simulink model "GTA_PCMFirmware"  (Simulink 7.8)
settings: Solver=FixedStepDiscrete  StartTime=0.0  StopTime=10.0  RelTol=1e-3
PreLoadFcn:
  | try, eval([bdroot '_setup']); catch, eval('model_setup', ''); end
InitFcn:
  | try, eval([bdroot '_setup']); catch, eval('model_setup', ''); end
undefined symbols (not defined in the file): fndFwd, fndNeut, fndRev, FWDlockout, GCM, keySwIgn2, motohawk_build_version, motohawk_trunc_name, motohawk_vardec_path, REVlockout
libraries: MotoHawk_lib x313, simulink x47, GTA_Library x13
(part 7 of 7)

== stateflow chart Function/2 Control Loop/Mode Control & Ready/Mode Control/Mode Control ==
  state ModeControl [parallel]
    settings: executionOrder=1
    state RUN
      state Drive
        en:
        ModeState = 5;
        HVmode = 3;
      state Startup
        en:
        ModeState = 0;
        HVmode = 0;
        ChargeEnable = 0;
      state Charge
        en:
        ModeState = 1;
        HVmode = 2;
        ChargeEnable = 1;
      state ChargeAndACC
        en:
        ModeState = 2;
        HVmode = 2;
        ChargeEnable = 1;
      state ACC1
        en:
        ModeState = 3;
        HVmode = 0;
        ChargeEnable = 0;
      state ACC2
        en:
        ModeState = 4;
        HVmode = 1;
      Startup -> Charge [order 1] : [acPresent == 1]
      (default) -> Startup
      Charge -> ChargeAndACC [order 1] : [keySw > 0]
      ChargeAndACC -> Charge [order 1] : [keySw == 0]
      Startup -> ACC1 [order 2] : [keySw > 0]
      ACC1 -> Startup [order 1] : [keySw == 0]
      ChargeAndACC -> ACC1 [order 2] : [acPresent == 0]
      ACC1 -> ChargeAndACC [order 2] : [acPresent == 1]
      ACC1 -> ACC2 [order 3] : [keySw > 1]
      ACC2 -> ACC1 [order 1] : [keySw < 2]
      ACC2 -> Drive [order 2] : [Ready == 1 && keySw == 6]
      Drive -> ACC1 [order 1] : [keySw < 2]
      ACC2 -> ChargeAndACC [order 3] : [acPresent == 1]
      Drive -> ChargeAndACC [order 2] : [acPresent == 1]
      Charge -> Startup [order 2] : [acPresent == 0]
    state Inhibit
      en:
      ModeState = 7;
      ChargeEnable = 0;
      HVmode = 0;
    RUN -> Inhibit : SysFault
    (default) -> RUN
  state HVControl [parallel]
    settings: executionOrder=2
    state Mode0
      en:
      HVstate = 0;
      SSCont = 0;
      MainCont = 0;
      HVaccRly = 0;
      DriveOn = 0;
    state DriveOn
      en:
      HVstate = 1;
      SSCont = 1;
      MainCont = 0;
      HVaccRly = 0;
      DriveOn = 0;
    state Limbo
    state PreCharge
      en:
      HVstate = 2;
      SSCont = 1;
      MainCont = 0;
      HVaccRly = 0;
      DriveOn = 1;
    state PreCharge2
      en:
      HVstate = 3;
      SSCont = 1;
      MainCont = 1;
      HVaccRly = 0;
      DriveOn = 1;
    state Mode1
      en:
      HVstate = 4;
      SSCont = 1;
      MainCont = 1;
      HVaccRly = 0;
      DriveOn = 0;
    state Mode3
      en:
      HVstate = 8;
      SSCont = 1;
      MainCont = 1;
      HVaccRly = 1;
      DriveOn = 1;
    state Mode2
      en:
      HVstate = 5;
      SSCont = 0;
      MainCont = 1;
      HVaccRly = 1;
      DriveOn = 0;
    state DriveDisable
      en:
      HVstate = 7;
      SSCont = 0;
      MainCont = 1;
      HVaccRly = 0;
      DriveOn = 0;
    state Startup_PauseHV
      en:
      HVstate = 0;
      SSCont = 0;
      MainCont = 0;
      HVaccRly = 0;
      DriveOn = 0
    Mode0 -> HVControl.DriveOn : [HVmode > 0]
    HVControl.DriveOn -> Mode0 [order 1] : [HVmode == 0]
    HVControl.DriveOn -> Limbo [order 2] : [VoltDiffPercent < 25]
    Limbo -> (junction 36) [order 1] : after(1000, tick) /send (ContFault);
    HVControl.DriveOn -> PreCharge [order 3] : after(100, tick)
    Limbo -> PreCharge [order 2] : [VoltDiffPercent > 25]
    (junction 37) -> (junction 36)
    PreCharge -> (junction 37) [order 1] : after(1000, tick) /send (PreChargeFault);
    PreCharge -> PreCharge2 [order 2] : [VoltDiffPercent < 25]
    PreCharge2 -> (junction 37) [order 1] : [HVmode == 0]
    (junction 36) -> Mode0
    PreCharge2 -> Mode1 [order 2] : [HVmode == 1]
    PreCharge2 -> Mode1 [order 3] : [HVmode == 2]
    PreCharge2 -> Mode3 [order 4] : [HVmode == 3]
    Mode1 -> Mode3 [order 1] : [HVmode == 3]
    Mode1 -> Mode2 [order 2] : [HVmode == 2]
    Mode2 -> Mode1 [order 1] : [HVmode == 1]
    Mode2 -> Mode3 [order 2] : [HVmode == 3]
    Mode3 -> Mode2 [order 2] : [HVmode < 3]
    Mode1 -> (junction 38) [order 3] : [HVmode == 0]
    Mode2 -> (junction 38) [order 3] : [HVmode == 0]
    (junction 38) -> DriveDisable
    DriveDisable -> (junction 39) : after(20,tick)
    PreCharge -> (junction 39) [order 3] : [HVmode == 0]
    (junction 39) -> Mode0
    Mode3 -> Mode1 [order 1] : [HVmode == 1]
    (default) -> Startup_PauseHV
    Startup_PauseHV -> Mode0 : after(100, tick)
  state FaultControl [parallel]
    settings: executionOrder=4
    state eStop_Fault
      en:
      Fault_ID = 1;
    state Battery_Fault
      en:
      Fault_ID = 2;
    state Contactor_Fault
      en:
      Fault_ID = 4;
    state Startup_Pause
      en:
      Fault_ID = 0;
    state PreCharge_Fault
      en:
      Fault_ID = 5;
    state HVOff
      en:
      Fault_ID = 0;
    state Fault_Send
    state Fault_Sent
    HVOff -> eStop_Fault [order 1] : after(600, tick) [eStop == 1]
    HVOff -> Battery_Fault [order 2] : [BatteryFault > 0 && ChargeEnable == 0]
    Contactor_Fault -> Fault_Send
    HVOff -> Contactor_Fault [order 4] : ContFault
    HVOff -> PreCharge_Fault [order 3] : PreChargeFault
    eStop_Fault -> Fault_Send
    Battery_Fault -> Fault_Send
    (default) -> Startup_Pause
    Startup_Pause -> HVOff : after(200,tick)
    PreCharge_Fault -> Fault_Send
    Fault_Send -> Fault_Sent : /send (SysFault);
  state DriveControl [parallel]
    settings: executionOrder=3
    state HVoff
      en:
      DriveState = 0;
      DriveEnable = 0;
      MotorEnable = 0;
    state DriveOn
      en:
      DriveState = 1;
      DriveEnable = 1;
      MotorEnable = 0;
    state RuneMode
      en:
      DriveState = 2;
      DriveEnable = 1;
      MotorEnable = 1;
    (default) -> HVoff
    HVoff -> DriveControl.DriveOn : [DriveOn ==1]
    DriveControl.DriveOn -> HVoff [order 1] : [DriveOn == 0]
    DriveControl.DriveOn -> RuneMode [order 2] : [ModeState == 5 && HVstate == 8]
    RuneMode -> DriveControl.DriveOn : [ModeState ~= 5 || HVstate < 8]
  data: SSCont output boolean; MainCont output boolean; DriveEnable output boolean; HVaccRly output boolean; ModeState output uint8; ChargeEnable output boolean; HVstate output uint8; Fault_ID output uint8; DriveState output uint8; MotorEnable output boolean; HVmode local uint8; DriveOn local boolean; Ready input boolean; VoltageFault input boolean; BatteryFault input boolean; keySw input uint8; eStop input boolean; acPresent input boolean; VoltDiffPercent input single
  events: PreChargeFault local EITHER_EDGE_EVENT; ContFault local EITHER_EDGE_EVENT; SysFault local EITHER_EDGE_EVENT

== stateflow chart Function/2 Control Loop/Component Controls/Body Control/Defroster/Chart ==
  state Defroster_Off
    en:
    Defrost=0;
  state Switch_Release
  state Wait
    Defrost=0;
  state Defroster_On
    en:
    Defrost=1;
  (default) -> Defroster_Off
  Defroster_Off -> Switch_Release : [Defrost_sw==1]
  Defroster_On -> Wait [order 2] : after(60000,tick)
  Defroster_On -> Switch_Release [order 1] : after(200,tick) [Defrost_sw==1]
  Wait -> Defroster_Off : [Defrost_sw==0]
  Switch_Release -> Defroster_On : after(10,tick) [Defrost_sw==0]
  data: Defrost output boolean size=1; Defrost_sw input boolean size=1

== stateflow chart Function/2 Control Loop/Component Controls/Body Control/Inter Wiper/Chart ==
  state Calc
    en:
    Wiper_out=0;
  state Output_On
    en:
    Wiper_out=1;
  state State
    en:
    Time=200+(50*Pot_position);
    PotHi=Pot_position + 5;
    PotLo=Pot_position - 5;
  state Wiper_reset
  state Output_Off
    en:
    Wiper_out=0;
  Calc -> Output_On : [Wiper_Enable==1]
  Output_On -> Output_Off : after(200,tick)
  (default) -> Calc
  State -> Calc [order 1] : after(Time,tick)
  State -> Calc [order 2] : [Wiper_Enable==0]
  State -> Wiper_reset [order 3] : after(100,tick)[(Pot_position < PotLo) | (Pot_position > PotHi)]
  Wiper_reset -> Output_On
  Output_Off -> State : after(100,tick)
  data: Wiper_out output boolean size=1; Pot_position input single size=1; Time local uint32 size=1; Wiper_Enable input boolean size=1; PotLo local uint32 size=1; PotHi local uint32 size=1

== stateflow chart Function/2 Control Loop/Component Controls/Display Control/Fault Lamps/Red ErrorCodes ==
  state Error_Start
    en:
    Count = 0;
    State = 0;
    Error_out = 0;
  state Error3_Check
    state Error_Off
      en:
      Error_out=0;
    state Error_on
      en:
      Error_out = 1;
      Count = Count +1;
    state Error_en
      en:
      Count = 0;
    state Done
      en:
      State=3;
    Error3_Check.Error_Off -> Error3_Check.Done [order 2] : [Count >= Error3_blinks]
    Error3_Check.Error_on -> Error3_Check.Error_Off : after(150, tick)
    Error3_Check.Error_Off -> Error3_Check.Error_on [order 1] : after(150,tick)
    Error3_Check.Error_en -> Error3_Check.Error_on [order 2] : [Error3 ==1]
    (default) -> Error3_Check.Error_en
    Error3_Check.Error_en -> Error3_Check.Done [order 1] : [Error3 == 0]
  state Error2_Check
    state Error_Off
      en:
      Error_out=0;
    state Done
      en:
      State=2;
    state Error_on
      en:
      Error_out = 1;
      Count = Count +1;
    state Error_en
      en:
      Count = 0;
    Error2_Check.Error_Off -> Error2_Check.Error_on [order 1] : after(150,tick)
    Error2_Check.Error_Off -> Error2_Check.Done [order 2] : [Count >= Error2_blinks]
    Error2_Check.Error_on -> Error2_Check.Error_Off : after(150, tick)
    Error2_Check.Error_en -> Error2_Check.Done [order 1] : [Error2 == 0]
    Error2_Check.Error_en -> Error2_Check.Error_on [order 2] : [Error2 ==1]
    (default) -> Error2_Check.Error_en
  state Error1_Check
    state Error_en
      en:
      Count = 0;
    state Done
      en:
      State=1;
    state Error_on
      en:
      Error_out = 1;
      Count = Count +1;
    state Error_Off
      en:
      Error_out=0;
    (default) -> Error1_Check.Error_en
    Error1_Check.Error_en -> Error1_Check.Done [order 1] : [Error1 == 0]
    Error1_Check.Error_en -> Error1_Check.Error_on [order 2] : [Error1 ==1]
    Error1_Check.Error_Off -> Error1_Check.Done [order 2] : [Count >= Error1_blinks]
    Error1_Check.Error_Off -> Error1_Check.Error_on [order 1] : after(150,tick)
    Error1_Check.Error_on -> Error1_Check.Error_Off : after(150, tick)
  state Wait
  state Wait1
  state Wait2
  (default) -> Error_Start
  Error_Start -> Error1_Check
  Error1_Check -> Wait : [State==1]
  Error3_Check -> Wait2 : [State==3]
  Error2_Check -> Wait1 : [State==2]
  Wait -> Error2_Check : after(500,tick)
  Wait1 -> Error3_Check : after(500,tick)
  Wait2 -> Error_Start : after(500,tick)
  data: Error1 input double; Error1_blinks input double; Error2 input double; Error2_blinks input double; Error3 input double; Error3_blinks input double; Count output double; State output double; Error_out output boolean

== stateflow chart Function/2 Control Loop/Component Controls/Display Control/Fault Lamps/Yellow ErrorCodes ==
  state Error_Start
    en:
    Count = 0;
    State = 0;
    Error_out = 0;
  state Error3_Check
    state Error_Off
      en:
      Error_out=0;
    state Error_on
      en:
      Error_out = 1;
      Count = Count +1;
    state Error_en
      en:
      Count = 0;
    state Done
      en:
      State=3;
    Error3_Check.Error_Off -> Error3_Check.Done [order 2] : [Count >= Error3_blinks]
    Error3_Check.Error_on -> Error3_Check.Error_Off : after(150, tick)
    Error3_Check.Error_Off -> Error3_Check.Error_on [order 1] : after(150,tick)
    Error3_Check.Error_en -> Error3_Check.Error_on [order 2] : [Error3 ==1]
    (default) -> Error3_Check.Error_en
    Error3_Check.Error_en -> Error3_Check.Done [order 1] : [Error3 == 0]
  state Error2_Check
    state Error_Off
      en:
      Error_out=0;
    state Done
      en:
      State=2;
    state Error_on
      en:
      Error_out = 1;
      Count = Count +1;
    state Error_en
      en:
      Count = 0;
    Error2_Check.Error_Off -> Error2_Check.Error_on [order 1] : after(150,tick)
    Error2_Check.Error_Off -> Error2_Check.Done [order 2] : [Count >= Error2_blinks]
    Error2_Check.Error_on -> Error2_Check.Error_Off : after(150, tick)
    Error2_Check.Error_en -> Error2_Check.Done [order 1] : [Error2 == 0]
    Error2_Check.Error_en -> Error2_Check.Error_on [order 2] : [Error2 ==1]
    (default) -> Error2_Check.Error_en
  state Error1_Check
    state Error_en
      en:
      Count = 0;
    state Done
      en:
      State=1;
    state Error_on
      en:
      Error_out = 1;
      Count = Count +1;
    state Error_Off
      en:
      Error_out=0;
    (default) -> Error1_Check.Error_en
    Error1_Check.Error_en -> Error1_Check.Done [order 1] : [Error1 == 0]
    Error1_Check.Error_en -> Error1_Check.Error_on [order 2] : [Error1 ==1]
    Error1_Check.Error_Off -> Error1_Check.Done [order 2] : [Count >= Error1_blinks]
    Error1_Check.Error_Off -> Error1_Check.Error_on [order 1] : after(150,tick)
    Error1_Check.Error_on -> Error1_Check.Error_Off : after(150, tick)
  state Wait
  state Wait1
  state Wait2
  (default) -> Error_Start
  Error_Start -> Error1_Check
  Error1_Check -> Wait : [State==1]
  Error3_Check -> Wait2 : [State==3]
  Error2_Check -> Wait1 : [State==2]
  Wait -> Error2_Check : after(500,tick)
  Wait1 -> Error3_Check : after(500,tick)
  Wait2 -> Error_Start : after(500,tick)
  data: Error1 input double; Error1_blinks input double; Error2 input double; Error2_blinks input double; Error3 input double; Error3_blinks input double; Count output double; State output double; Error_out output boolean

== stateflow chart Function/2 Control Loop/Component Controls/Motor Control/Direction Selector & Control Loop/Rate Limiter Control Loop ==
  state Start
    Current_Out=0;
    ErrorAccum=0;
  state Error_calc
    error=Current_In - Current_Feedback;
  state Rising
    Current_Out = Current_Feedback + Rise;
  state Falling
    Current_Out = Current_Feedback + Fall;
  state Target
    Current_Out = Current_In;
  (default) -> Start
  Start -> Error_calc [order 2]
  Error_calc -> Rising [order 2] : [error > Rise]
  Error_calc -> Falling [order 3] : [error < Fall]
  Error_calc -> Target [order 4]
  Target -> Error_calc
  Rising -> Error_calc
  Falling -> Error_calc
  Start -> Start [order 1] : [Fall >= 0 || Rise <=0]
  Error_calc -> Start [order 1] : [Fall >= 0 || Rise <=0]
  data: Current_In input double; Current_Feedback input double; Current_Out output double; error local double; Rise input double; Fall input double; ErrorAccum local double
